simulink model "parallelForcePosition"  (R2021a)
settings: Solver=VariableStepAuto  StartTime=0.0  StopTime=15  RelTol=1e-3
values from neighbouring files (symbols this model uses):
  C_f_P = K_f    [assignment15_main.m]
  f_d = [0 -0.5 0 0 0 0].'    [assignment15_main.m]
  K = diag([0 10 0 10 0 0])    [assignment15_main.m]
  K_f = 0.3*diag([10 10 10 10 10 10])    [assignment15_main.m]
  K_i = 0.1*diag([10 10 10 10 10 10])    [assignment15_main.m]
  Kd = 20*diag([10 10 10 10 10 10])    [assignment15_main.m]
  Kp = 50*diag([10 10 10 10 10 10])    [assignment15_main.m]
  M_d = 0.1*diag([10 10 10 10 10 10])    [assignment15_main.m]
  x_d = [0 -0.3 0.6 pi/2 -pi/2 0].'    [assignment15_main.m]
libraries: vrlib x1
settings Model: Creator=fabio  LastModifiedBy=fabio

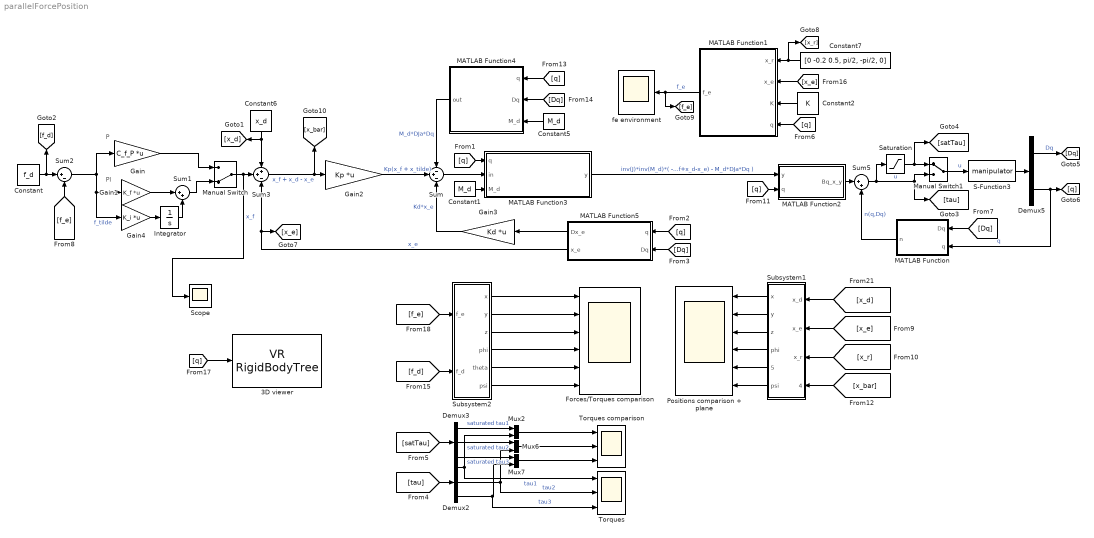
== system parallelForcePosition ==
  note: PI
  note: P
  3D viewer : vrlib/VR RigidBodyTree  RBT=robot  useRBT=off  Ts=0.5  ForceViewerOpen=on
      settings: SourceProductBaseCode=SL
  Constant : Constant  Value=f_d
  Constant1 : Constant  Value=M_d  VectorParams1D=off
  Constant2 : Constant  Value=K  VectorParams1D=off
  Constant5 : Constant  Value=M_d  VectorParams1D=off
  Constant6 : Constant  Value=x_d
  Constant7 : Constant  Value=[0 -0.2 0.5, pi/2, -pi/2, 0]
  Demux2 : Demux  Outputs=3
  Demux3 : Demux  Outputs=3
  Demux5 : Demux  Outputs=[3 3]
  Forces/Torques comparison : Scope  NumInputPorts=6
  Gain : Gain  Gain=C_f_P  Multiplication=Matrix(K*u)
  Gain1 : Gain  Gain=K_f  Multiplication=Matrix(K*u)
  Gain2 : Gain  Gain=Kp  Multiplication=Matrix(K*u) (u vector)
  Gain3 : Gain  Gain=Kd  Multiplication=Matrix(K*u) (u vector)
  Gain4 : Gain  Gain=K_i  Multiplication=Matrix(K*u)
  Integrator : Integrator
  MATLAB Function : MATLAB Function  TreatAsAtomicUnit=on
  MATLAB Function1 : MATLAB Function  TreatAsAtomicUnit=on
  MATLAB Function2 : MATLAB Function  TreatAsAtomicUnit=on
  MATLAB Function3 : MATLAB Function  TreatAsAtomicUnit=on
  MATLAB Function4 : MATLAB Function  TreatAsAtomicUnit=on
  MATLAB Function5 : MATLAB Function  TreatAsAtomicUnit=on
  Manual Switch : ManualSwitch  CurrentSetting=0
  Manual Switch1 : ManualSwitch
  Mux2 : Mux  Inputs=2
  Mux6 : Mux  Inputs=2
  Mux7 : Mux  Inputs=2
  Positions comparison + plane : Scope  NumInputPorts=6
  S-Function3 : S-Function  FunctionName=manipulator  Parameters=myRobot  SFunctionDeploymentMode=off  EnableBusSupport=off
  Saturation : Saturate  UpperLimit=20  LowerLimit=-20
  Scope : Scope
  Subsystem1 : Subsystem
  Subsystem2 : Subsystem
  Sum : Sum  Inputs=-+-
  Sum1 : Sum  Inputs=|++
  Sum2 : Sum  Inputs=|+-
  Sum3 : Sum  Inputs=++-
  Sum5 : Sum  Inputs=|++
  Torques : Scope  NumInputPorts=3
  Torques comparison : Scope  NumInputPorts=3
  fe environment : Scope
  wires:
  Manual Switch1/1 -> S-Function3/1  "u"
  Sum3/1 -> [x_bar], Gain2/1  "x_f + x_d - x_e"
  S-Function3/1 -> Demux5/1
  Demux5/1 -> [Dq]  "Dq"
  Demux5/2 -> [q], MATLAB Function/2(q)  "q"
  Gain2/1 -> Sum/2  "Kp(x_f + x_tilde)"
  Sum/1 -> MATLAB Function3/2(in)
  MATLAB Function2/1(Bq_x_y) -> Sum5/1
  Demux2/1 -> Torques/1, Mux2/2  "tau1"
  [tau] -> Demux2/1
  Saturation/1 -> [satTau], Manual Switch1/1
  [satTau] -> Demux3/1
  Demux3/1 -> Mux2/1  "saturated tau1"
  Mux2/1 -> Torques comparison/1
  Mux6/1 -> Torques comparison/2
  Mux7/1 -> Torques comparison/3
  Demux2/2 -> Torques/2, Mux6/2  "tau2"
  Demux3/2 -> Mux6/1  "saturated tau2"
  Demux3/3 -> Mux7/1  "saturated tau3"
  Demux2/3 -> Torques/3, Mux7/2  "tau3"
  Sum5/1 -> [tau], Manual Switch1/2, Saturation/1  "u"
  MATLAB Function5/2(x_e) -> Sum3/3, [x_e]  "x_e"
  [Dq] -> MATLAB Function/1(Dq)
  [q] -> MATLAB Function2/2(q)
  [q] -> 3D viewer/1
  [q] -> MATLAB Function3/1(q)
  MATLAB Function3/1(y) -> MATLAB Function2/1(y)  "inv(J)*inv(M_d)*( -Kd*Dx_e + Kp*(x_f+x_d-x_e) - M_d*DJa*Dq )"
  [q] -> MATLAB Function5/1(q)
  [Dq] -> MATLAB Function5/2(Dq)
  MATLAB Function5/1(Dx_e) -> Gain3/1
  Gain3/1 -> Sum/3  "Kd*x_e"
  MATLAB Function4/1(out) -> Sum/1  "M_d*DJa*Dq"
  Constant7/1 -> MATLAB Function1/1(x_r), [x_r]
  [x_e] -> MATLAB Function1/2(x_e)
  Constant2/1 -> MATLAB Function1/3(K)
  MATLAB Function/1(n) -> Sum5/2  "n(q,Dq)"
  MATLAB Function1/1(f_e) -> fe environment/1, [f_e]  "f_e"
  [q] -> MATLAB Function1/4(q)
  [f_e] -> Sum2/2
  Constant1/1 -> MATLAB Function3/3(M_d)
  Constant/1 -> Sum2/1, [f_d]
  Constant6/1 -> Sum3/1, [x_d]
  Sum2/1 -> Gain4/1, Gain1/1, Gain/1  "f_tilde"
  Gain/1 -> Manual Switch/1
  Manual Switch/1 -> Scope/1, Sum3/2  "x_f"
  Gain4/1 -> Integrator/1
  Integrator/1 -> Sum1/2
  Sum1/1 -> Manual Switch/2
  Gain1/1 -> Sum1/1
  Constant5/1 -> MATLAB Function4/3(M_d)
  [Dq] -> MATLAB Function4/2(Dq)
  [q] -> MATLAB Function4/1(q)
  Subsystem1/4(phi) -> Positions comparison + plane/4
  [x_r] -> Subsystem1/3(x_r)
  Subsystem1/2(y) -> Positions comparison + plane/2
  [x_d] -> Subsystem1/1(x_d)
  Subsystem1/3(z) -> Positions comparison + plane/3
  Subsystem1/6(psi) -> Positions comparison + plane/6
  Subsystem1/1(x) -> Positions comparison + plane/1
  [x_e] -> Subsystem1/2(x_e)
  Subsystem1/5(theta) -> Positions comparison + plane/5
  [f_e] -> Subsystem2/1(f_e)
  Subsystem2/1(x) -> Forces/Torques comparison/1
  Subsystem2/2(y) -> Forces/Torques comparison/2
  Subsystem2/3(z) -> Forces/Torques comparison/3
  Subsystem2/4(phi) -> Forces/Torques comparison/4
  Subsystem2/5(theta) -> Forces/Torques comparison/5
  Subsystem2/6(psi) -> Forces/Torques comparison/6
  [f_d] -> Subsystem2/2(f_d)
  [x_bar] -> Subsystem1/4(x_bar)

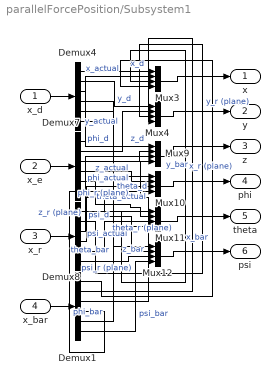
== system parallelForcePosition/Subsystem1 ==
  x_d : Inport
  x_e : Inport  Port=2
  x_r : Inport  Port=3
  x_bar : Inport  Port=4
  Demux{1,4,7..8} (4 alike) : Demux  Outputs=6
  Mux{3..4,9..12} (6 alike) : Mux
  x : Outport
  y : Outport  Port=2
  z : Outport  Port=3
  phi : Outport  Port=4
  theta : Outport  Port=5
  psi : Outport  Port=6
  wires:
  Demux8/1 -> Mux3/3  "x_r (plane)"
  Demux7/3 -> Mux9/2  "z_actual"
  Demux4/4 -> Mux10/1  "phi_d"
  Demux8/2 -> Mux4/3  "y_r (plane)"
  Demux7/6 -> Mux12/2  "psi_actual"
  Demux7/4 -> Mux10/2  "phi_actual"
  Demux7/1 -> Mux3/2  "x_actual"
  Demux8/3 -> Mux9/3  "z_r (plane)"
  Demux4/3 -> Mux9/1  "z_d"
  Demux4/6 -> Mux12/1  "psi_d"
  Demux4/5 -> Mux11/1  "theta_d"
  Demux7/5 -> Mux11/2  "theta_actual"
  Demux4/2 -> Mux4/1  "y_d"
  Demux4/1 -> Mux3/1  "x_d"
  Demux7/2 -> Mux4/2  "y_actual"
  Demux8/6 -> Mux12/3  "psi_r (plane)"
  Demux8/4 -> Mux10/3  "phi_r (plane)"
  Mux11/1 -> theta/1
  Demux8/5 -> Mux11/3  "theta_r (plane)"
  x_d/1 -> Demux4/1
  x_e/1 -> Demux7/1
  Mux9/1 -> z/1
  Mux12/1 -> psi/1
  Mux10/1 -> phi/1
  Mux4/1 -> y/1
  Mux3/1 -> x/1
  x_r/1 -> Demux8/1
  x_bar/1 -> Demux1/1
  Demux1/1 -> Mux3/4  "x_bar"
  Demux1/2 -> Mux4/4  "y_bar"
  Demux1/4 -> Mux10/4  "phi_bar"
  Demux1/3 -> Mux9/4  "z_bar"
  Demux1/5 -> Mux11/4  "theta_bar"
  Demux1/6 -> Mux12/4  "psi_bar"

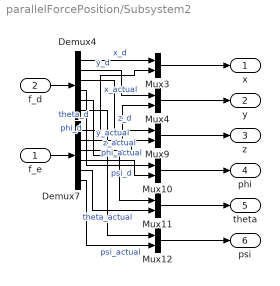
== system parallelForcePosition/Subsystem2 ==
  f_e : Inport
  f_d : Inport  Port=2
  Demux4 : Demux  Outputs=6
  Demux7 : Demux  Outputs=6
  Mux{3..4,9..12} (6 alike) : Mux  Inputs=2
  x : Outport
  y : Outport  Port=2
  z : Outport  Port=3
  phi : Outport  Port=4
  theta : Outport  Port=5
  psi : Outport  Port=6
  wires:
  Demux7/3 -> Mux9/2  "z_actual"
  Demux4/4 -> Mux10/1  "phi_d"
  Demux7/6 -> Mux12/2  "psi_actual"
  Demux7/4 -> Mux10/2  "phi_actual"
  Demux7/1 -> Mux3/2  "x_actual"
  Demux4/3 -> Mux9/1  "z_d"
  Demux4/6 -> Mux12/1  "psi_d"
  Demux4/5 -> Mux11/1  "theta_d"
  Demux7/5 -> Mux11/2  "theta_actual"
  Demux4/2 -> Mux4/1  "y_d"
  Demux4/1 -> Mux3/1  "x_d"
  Demux7/2 -> Mux4/2  "y_actual"
  Mux11/1 -> theta/1
  f_d/1 -> Demux4/1
  f_e/1 -> Demux7/1
  Mux9/1 -> z/1
  Mux12/1 -> psi/1
  Mux10/1 -> phi/1
  Mux4/1 -> y/1
  Mux3/1 -> x/1

== matlab function parallelForcePosition/MATLAB Function1 ==
  data: x_r input; x_e input; K input; f_e output; q input
function f_e  = environment(x_r, x_e, K, q)    
    
    y_plane = x_r(2);
    
    %contact with the plane
    if max(size(x_e)) > 1 && x_e(2) < y_plane
        f_e = K*(x_e - x_r);
    else %no contact with the plane
        f_e = [0 0 0 0 0 0].';
    end   
    
    %Get Ja from ∑0 to ∑ee
    if max(size(q)) < 3
        q = [0 0 0];   
    end    
end

== matlab function parallelForcePosition/MATLAB Function ==
  data: Dq input; n output; q input
function n = n_q_Dq(Dq, q)
    
    %To get the "perfect" matrices use the following code
    C = get_C_matrix(q,Dq);
    G = get_G_matrix(q);
    
    
    %To get the "wrongly estimated" matrices use the following code   
%     theta2 = q(2);   d3 = q(3); 
%     Dtheta2 = Dq(2); Dd3 = Dq(3); 
%     
%     m_Link4 = 0.16;  %0.2kg is the correct value
% 
%     C = [0,                         0,                        0;
%          0,            m_Link4*Dd3*d3,       m_Link4*Dtheta2*d3;
%          0,       -m_Link4*Dtheta2*d3,                        0];
%    
%     G = [           0                           ;
%          (981*m_Link4*sin(theta2)*d3)/100 ;
%           -(981*m_Link4*cos(theta2))/100    ];


    
    n = C*Dq + G; %F = friction is neglected

end

== matlab function parallelForcePosition/MATLAB Function2 ==
  data: y input; Bq_x_y output; q input
function Bq_x_y = Bq_x_y(y,q)
    Bq_x_y = get_B_matrix(q)*y;
end

== matlab function parallelForcePosition/MATLAB Function3 ==
  data: q input; y output; in input; M_d input
function y = invJa_x_invMd_x_in(q, in, M_d)
    if max(size(q)) < 3
        q = [0 0 0];   
    end
    
    Ja = get_Ja_matrix(q);    
    y = pinv(Ja) * pinv(M_d) * in;
 
end

== matlab function parallelForcePosition/MATLAB Function4 ==
  data: q input; out output; Dq input; M_d input
function out = M_d_x_DJa_x_Dq(q, Dq, M_d)
    if max(size(q)) < 3
        q = [0 0 0];   
    end
    if max(size(Dq)) < 3
        Dq = [0 0 0];   
    end
    
    %Get DJa from ∑0 to ∑ee 
    DJa = get_DJa_matrix(q, Dq);

    out = M_d * DJa * Dq;
      
end

== matlab function parallelForcePosition/MATLAB Function5 ==
  data: Dx_e output; q input; x_e output; Dq input
function [Dx_e, x_e] = k(q, Dq) 
     %Compute the direct kinematics from last transformation matrix
    if max(size(q)) < 3
        q = [0 0 0];   
    end
    if max(size(Dq)) < 3
        Dq = [0 0 0];   
    end
    
    %get rotation matrix and translation vector from ∑0 to ∑ee   
    T0_to_ee = get_T0_ee_matrix(q);
    R0_to_ee = T0_to_ee(1:3,1:3);
    p0_to_ee = T0_to_ee(1:3,4);    
                 
    eulerAngles = rotm2eul(R0_to_ee, 'ZYZ');
    
    x_e = [ p0_to_ee;
          eulerAngles.' ]; %return complete direct kinematics
      
    Ja = get_Ja_matrix(q);
    Dx_e = Ja * Dq;
end
